simulink model "EKFSim"  (R2020a)
settings: Solver=VariableStepAuto  StartTime=0.0  StopTime=37500  RelTol=1e-3
undefined symbols (not defined in the file or in its folder): sigbuilder_block
libraries: fl_lib x14, nesl_utility x14
settings Model: Creator=WL  LastModifiedBy=Marvin
settings DataIOCC: ReturnWorkspaceOutputs=off
settings DebuggingCC: ArithmeticOperatorsInVariantConditions=warning
settings SFSimCC: SimUseLocalCustomCode=off  CustomCodeUndefinedFunction=UseInterfaceOnly
settings RTWCC: RTWUseLocalCustomCode=off
settings CodeAppCC: StateflowObjectComments=on

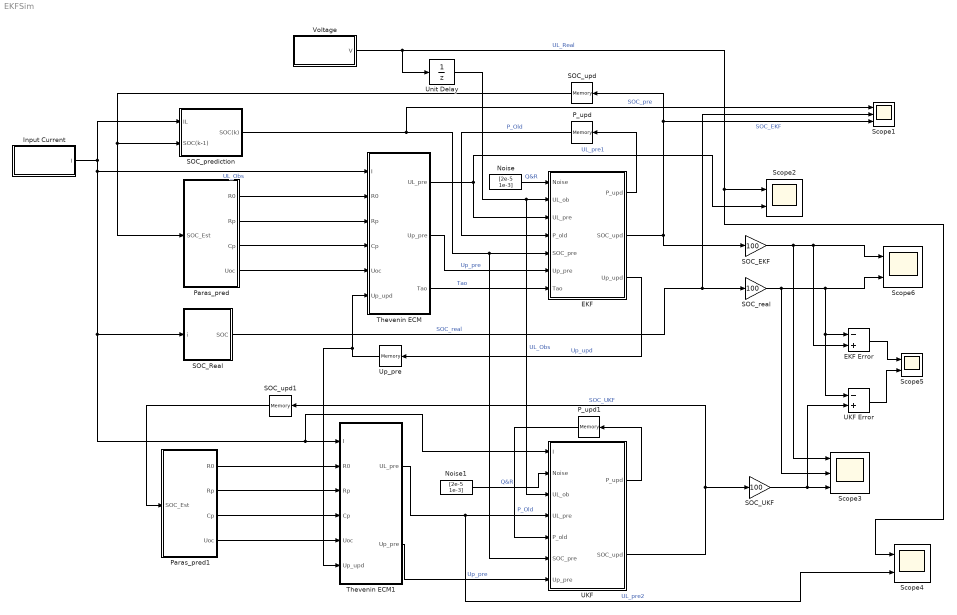
== system EKFSim ==
  EKF : MATLAB Function  TreatAsAtomicUnit=on
  EKF Error : Sum  Inputs=-+
  Input Current : Subsystem  Tag=STV Subsys  LoadFcn=sigbuilder_block('load');  StartFcn=sigbuilder_block('start');  StopFcn=sigbuilder_block('stop');  ClipboardFcn=sigbuilder_block('clipboard');  mask(Sigbuilder block){tuvar=[0:10]}
      mask help: Simulink:masks:SigbuilderBlock_MD
      mask init:
      | if ~strcmp(get_param(bdroot(gcbh),'SimulationStatus'),'stopped') tuvar = sigbuilder_block('maskInit'); end
      settings: CopyFcn=sigbuilder_block('copy');  DeleteFcn=sigbuilder_block('delete');  ModelCloseFcn=sigbuilder_block('modelClose');  PreSaveFcn=sigbuilder_block('preSave');  PauseFcn=sigbuilder_block('pause');  ContinueFcn=sigbuilder_block('continue');  NameChangeFcn=sigbuilder_block('namechange');  OpenFcn=sigbuilder_block('open',[6 51 1012.5 460.5 ]);  CloseFcn=sigbuilder_block('close');
      mask Display: plot(0, 0, 100, 100,[2, 2, 32, 32, 2], [68, 8, 8, 68, 68],[32, 2], [38, 38], [32, 19, 2],[53, 60, 44], [32, 17, 17, 2],[16, 16, 31, 31]);txt = getActiveGroup(gcbh);text(2, 100, txt,'verticalAlignment', 'top');
  Noise : Constant  Value=[2e-5 1e-3]
  Noise1 : Constant  Value=[2e-5 1e-3]
  P_upd : Memory  InitialCondition=[0.02 0 0 0.01]  InheritSampleTime=on  LinearizeAsDelay=on
  P_upd1 : Memory  InitialCondition=[1e-6 1e-6]  InheritSampleTime=on  LinearizeAsDelay=on
  Paras_pred : Subsystem
  Paras_pred1 : Subsystem
  SOC_EKF : Gain  Gain=100
  SOC_Real : Subsystem
  SOC_UKF : Gain  Gain=100
  SOC_prediction : Subsystem
  SOC_real : Gain  Gain=100
  SOC_upd : Memory  InitialCondition=1  InheritSampleTime=on  LinearizeAsDelay=on
  SOC_upd1 : Memory  InitialCondition=1  InheritSampleTime=on  LinearizeAsDelay=on
  Scope1 : Scope  NumInputPorts=3
  Scope{2,4..6} (4 alike) : Scope  NumInputPorts=2
  Scope3 : Scope  NumInputPorts=3
  Thevenin ECM : Subsystem
  Thevenin ECM1 : Subsystem
  UKF : MATLAB Function  TreatAsAtomicUnit=on
  UKF Error : Sum  Inputs=-+
  Unit Delay : UnitDelay  InitialCondition=4.1912  SampleTime=0.1  HasFrameUpgradeWarning=on
  Up_pre : Memory  InheritSampleTime=on  LinearizeAsDelay=on
  "Voltage " : Subsystem  Tag=STV Subsys  LoadFcn=sigbuilder_block('load');  StartFcn=sigbuilder_block('start');  StopFcn=sigbuilder_block('stop');  ClipboardFcn=sigbuilder_block('clipboard');  mask(Sigbuilder block){tuvar=[0:10]}
      mask help: Simulink:masks:SigbuilderBlock_MD
      mask init:
      | if ~strcmp(get_param(bdroot(gcbh),'SimulationStatus'),'stopped') tuvar = sigbuilder_block('maskInit'); end
      settings: CopyFcn=sigbuilder_block('copy');  DeleteFcn=sigbuilder_block('delete');  ModelCloseFcn=sigbuilder_block('modelClose');  PreSaveFcn=sigbuilder_block('preSave');  PauseFcn=sigbuilder_block('pause');  ContinueFcn=sigbuilder_block('continue');  NameChangeFcn=sigbuilder_block('namechange');  OpenFcn=sigbuilder_block('open',[6 51 1012.5 460.5 ]);  CloseFcn=sigbuilder_block('close');
      mask Display: plot(0, 0, 100, 100,[2, 2, 32, 32, 2], [68, 8, 8, 68, 68],[32, 2], [38, 38], [32, 19, 2],[53, 60, 44], [32, 17, 17, 2],[16, 16, 31, 31]);txt = getActiveGroup(gcbh);text(2, 100, txt,'verticalAlignment', 'top');
  wires:
  Paras_pred/4(Uoc) -> Thevenin ECM/5(Uoc)
  Paras_pred/1(R0) -> Thevenin ECM/2(R0)
  Paras_pred/3(Cp) -> Thevenin ECM/4(Cp)
  Paras_pred/2(Rp) -> Thevenin ECM/3(Rp)
  Thevenin ECM/1(UL_pre) -> Scope2/2, EKF/3(UL_pre)  "UL_pre1"
  "Voltage "/1(V) -> Unit Delay/1, Scope2/1, Scope4/1  "UL_Real"
  Thevenin ECM/2(Up_pre) -> EKF/6(Up_pre)  "Up_pre"
  Noise/1 -> EKF/1(Noise)  "Q&R"
  SOC_prediction/1(SOC(k)) -> Scope1/1, EKF/5(SOC_pre), UKF/6(SOC_pre)  "SOC_pre"
  P_upd/1 -> EKF/4(P_old)  "P_Old"
  SOC_upd/1 -> Paras_pred/1(SOC_Est), SOC_prediction/2(SOC(k-1))
  EKF/1(P_upd) -> P_upd/1
  Thevenin ECM/3(Tao) -> EKF/7(Tao)  "Tao"
  EKF/3(Up_upd) -> Up_pre/1  "Up_upd"
  Up_pre/1 -> Thevenin ECM1/6(Up_upd), Thevenin ECM/6(Up_upd)
  EKF/2(SOC_upd) -> SOC_EKF/1, Scope1/3, SOC_upd/1  "SOC_EKF"
  Unit Delay/1 -> UKF/3(UL_ob), EKF/2(UL_ob)  "UL_Obs"
  EKF Error/1 -> Scope5/1
  Noise1/1 -> UKF/2(Noise)  "Q&R"
  UKF/1(P_upd) -> P_upd1/1
  P_upd1/1 -> UKF/5(P_old)  "P_Old"
  Thevenin ECM1/1(UL_pre) -> Scope4/2, UKF/4(UL_pre)  "UL_pre2"
  Thevenin ECM1/2(Up_pre) -> UKF/7(Up_pre)  "Up_pre"
  UKF/2(SOC_upd) -> SOC_UKF/1, SOC_upd1/1  "SOC_UKF"
  Paras_pred1/1(R0) -> Thevenin ECM1/2(R0)
  Paras_pred1/2(Rp) -> Thevenin ECM1/3(Rp)
  Paras_pred1/3(Cp) -> Thevenin ECM1/4(Cp)
  Paras_pred1/4(Uoc) -> Thevenin ECM1/5(Uoc)
  SOC_upd1/1 -> Paras_pred1/1(SOC_Est)
  Input Current/1(I) -> SOC_Real/1(i), UKF/1(I), Thevenin ECM1/1(I), Thevenin ECM/1(I), SOC_prediction/1(IL)  "UL_Obs"
  SOC_Real/1(SOC) -> Scope1/2, SOC_real/1  "SOC_real"
  SOC_EKF/1 -> Scope6/1, EKF Error/2, Scope3/1
  SOC_real/1 -> Scope3/2, Scope6/2, UKF Error/1, EKF Error/1
  SOC_UKF/1 -> UKF Error/2, Scope3/3
  UKF Error/1 -> Scope5/2

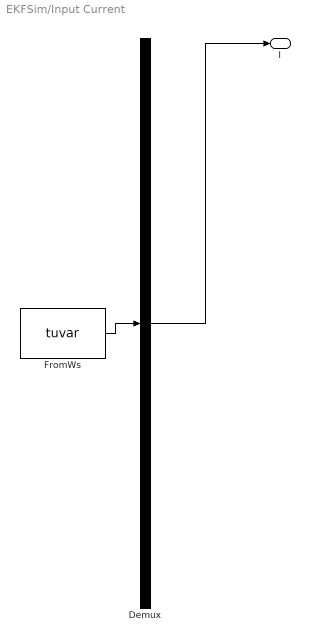
== system EKFSim/Input Current ==
  Demux : Demux  Tag=STV Demux  Outputs=1
      settings: DisplayOption=none
  FromWs : FromWorkspace  Tag=STV FromWs  VariableName=tuvar
      SigBuilderData=|
      | common.afterFinalStr = 'Extrapolate'
      | common.sampleTime = 0
      | dataSet.timeRange = [0 37520]
      | dataSet.name = 'Sheet1'
      | sbobj.Name = 'Signal Builder'
      | sbobj.Groups.Name = 'Sheet1'
      | sbobj.Groups.Signals.Name = 'I'
      | sbobj.Groups.Signals.XData = [0 1.01353925251 2.02707850502 3.04061775753 8.33038044522 13.6201431329 18.9099058206 24.1996685083 30.9141105575 35.6042291656 40.2943477737 44.9844663818 ... (4125 elements, 1x4125)]
      | sbobj.Groups.Signals.YData = [0.089857 0.0908255381097 0.0917940762194 0.0927626143291 0.0978175115535 0.0992265626287 0.0989541398502 0.0981051025856 0.1 0.0879771034309 0.0809245842985 0.0814437804285 ... (4125 elements, 1x4125)]
      | sbobj.Groups.TimeRange = [0 37520]
  I : Outport  VectorParamsAs1DForOutWhenUnconnected=off
  wires:
  Demux/1 -> I/1
  FromWs/1 -> Demux/1

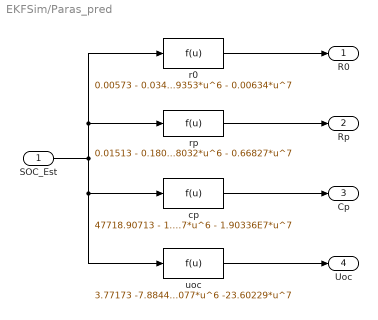
== system EKFSim/Paras_pred ==
  SOC_Est : Inport
  cp : Fcn  Expr=47718.90713 - 1.00583E6*u^1 + 9.2653E6*u^2 - 3.91088E7*u^3 + 8.85892E7*u^4 - 1.11014E8*u^5 + 7.22811E7*u^6 - 1.90336E7*u^7
  r0 : Fcn  Expr=0.00573 - 0.03427*u^1 + 0.1455*u^2 - 0.32647*u^3 + 0.41465*u^4 - 0.28992*u^5 + 0.09353*u^6 - 0.00634*u^7
  rp : Fcn  Expr=0.01513 - 0.18008*u^1 + 1.05147*u^2 - 3.27616*u^3 + 5.79793*u^4 - 5.81819*u^5 + 3.08032*u^6 - 0.66827*u^7
  uoc : Fcn  Expr=3.77173 -7.88447*u^1 + 60.21383*u^2 -200.15462*u^3 + 345.34531*u^4 - 314.92282*u^5 + 141.34077*u^6 -23.60229*u^7
  R0 : Outport  VectorParamsAs1DForOutWhenUnconnected=off
  Rp : Outport  Port=2  VectorParamsAs1DForOutWhenUnconnected=off
  Cp : Outport  Port=3  VectorParamsAs1DForOutWhenUnconnected=off
  Uoc : Outport  Port=4  VectorParamsAs1DForOutWhenUnconnected=off
  wires:
  cp/1 -> Cp/1
  rp/1 -> Rp/1
  uoc/1 -> Uoc/1
  r0/1 -> R0/1
  SOC_Est/1 -> uoc/1, cp/1, rp/1, r0/1

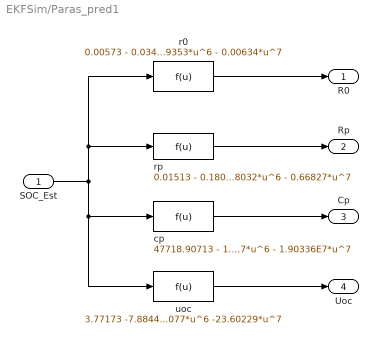
== system EKFSim/Paras_pred1 ==
  SOC_Est : Inport
  cp : Fcn  Expr=47718.90713 - 1.00583E6*u^1 + 9.2653E6*u^2 - 3.91088E7*u^3 + 8.85892E7*u^4 - 1.11014E8*u^5 + 7.22811E7*u^6 - 1.90336E7*u^7
  r0 : Fcn  Expr=0.00573 - 0.03427*u^1 + 0.1455*u^2 - 0.32647*u^3 + 0.41465*u^4 - 0.28992*u^5 + 0.09353*u^6 - 0.00634*u^7
  rp : Fcn  Expr=0.01513 - 0.18008*u^1 + 1.05147*u^2 - 3.27616*u^3 + 5.79793*u^4 - 5.81819*u^5 + 3.08032*u^6 - 0.66827*u^7
  uoc : Fcn  Expr=3.77173 -7.88447*u^1 + 60.21383*u^2 -200.15462*u^3 + 345.34531*u^4 - 314.92282*u^5 + 141.34077*u^6 -23.60229*u^7
  R0 : Outport  VectorParamsAs1DForOutWhenUnconnected=off
  Rp : Outport  Port=2  VectorParamsAs1DForOutWhenUnconnected=off
  Cp : Outport  Port=3  VectorParamsAs1DForOutWhenUnconnected=off
  Uoc : Outport  Port=4  VectorParamsAs1DForOutWhenUnconnected=off
  wires:
  cp/1 -> Cp/1
  rp/1 -> Rp/1
  uoc/1 -> Uoc/1
  SOC_Est/1 -> uoc/1, cp/1, r0/1, rp/1
  r0/1 -> R0/1

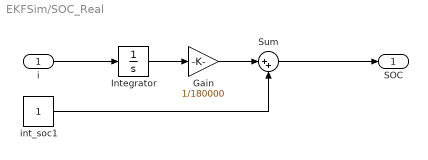
== system EKFSim/SOC_Real ==
  i : Inport
  Gain : Gain  Gain=1/180000
  Integrator : Integrator
  Sum : Sum  Inputs=|++
  int_soc1 : Constant
  SOC : Outport  VectorParamsAs1DForOutWhenUnconnected=off
  wires:
  Gain/1 -> Sum/1
  Integrator/1 -> Gain/1
  int_soc1/1 -> Sum/2
  i/1 -> Integrator/1
  Sum/1 -> SOC/1

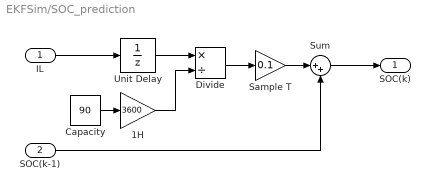
== system EKFSim/SOC_prediction ==
  IL : Inport
  SOC(k-1) : Inport  Port=2
  1H : Gain  Gain=3600
  Capacity : Constant  Value=90
  Divide : Product  Inputs=*/
  Sample T : Gain  Gain=0.1
  Sum : Sum  Inputs=|++
  Unit Delay : UnitDelay  SampleTime=0.15  HasFrameUpgradeWarning=on
  SOC(k) : Outport  VectorParamsAs1DForOutWhenUnconnected=off
  wires:
  Sample T/1 -> Sum/1
  Unit Delay/1 -> Divide/1
  SOC(k-1)/1 -> Sum/2
  IL/1 -> Unit Delay/1
  Sum/1 -> SOC(k)/1
  Capacity/1 -> 1H/1
  1H/1 -> Divide/2
  Divide/1 -> Sample T/1

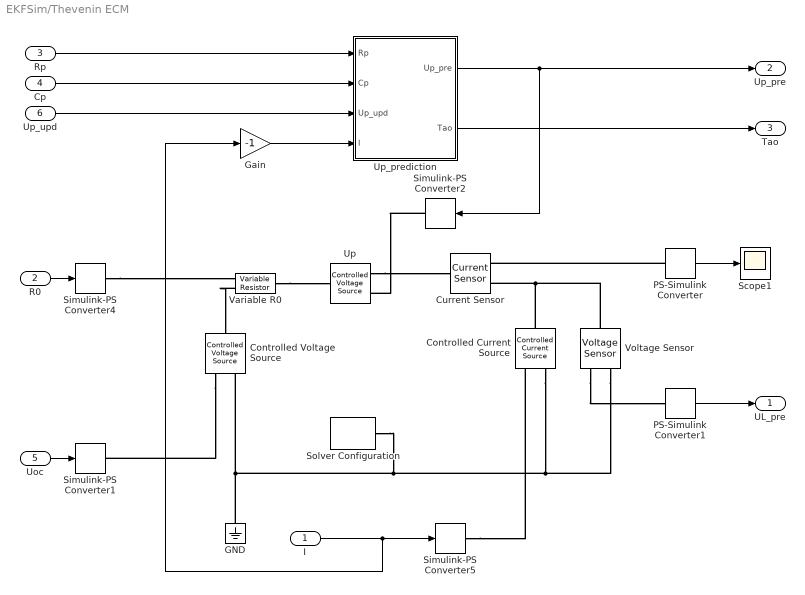
== system EKFSim/Thevenin ECM ==
  I : Inport
  R0 : Inport  Port=2
  Rp : Inport  Port=3
  Cp : Inport  Port=4
  Uoc : Inport  Port=5
  Up_upd : Inport  Port=6
  Controlled Current Source : fl_lib/Electrical/Electrical Sources/Controlled Current Source
  Controlled Voltage Source : fl_lib/Electrical/Electrical Sources/Controlled Voltage Source
  Current Sensor : fl_lib/Electrical/Electrical Sensors/Current Sensor
  GND : fl_lib/Electrical/Electrical Elements/Electrical Reference
  Gain : Gain  Gain=-1
  PS-Simulink Converter : nesl_utility/PS-Simulink Converter  PhysicalDomain=network_engine_domain  SubClassName=ps_output  LeftPortType=input  RightPortType=output  PseudoPeriodic=off  Frequencies=[]  Unit=A  AffineConversion=off
  PS-Simulink Converter1 : nesl_utility/PS-Simulink Converter  PhysicalDomain=network_engine_domain  SubClassName=ps_output  LeftPortType=input  RightPortType=output  PseudoPeriodic=off  Frequencies=[]  Unit=V  AffineConversion=off
  Scope1 : Scope
  Simulink-PS Converter{1..2,4..5} (4 alike) : nesl_utility/Simulink-PS Converter  PhysicalDomain=network_engine_domain  SubClassName=ps_input  LeftPortType=input  RightPortType=output  PseudoPeriodic=off  Frequencies=[]  NoiseDistribution=none  NoiseParameters=[]  Unit=1  AffineConversion=off  FilteringAndDerivatives=zero  SimscapeFilterOrder=1  InputFilterTimeConstant=0.001  UdotUserProvided=0
  Solver Configuration : nesl_utility/Solver Configuration  PhysicalDomain=network_engine_domain  SubClassName=solver  LeftPortType=input  RightPortType=generic  Tones=[]  Harmonics=[]  SimulateNoise=off  Profile=off  UseLocalSampling=off  EnableSwitchedLinearOptims=on  FrequencyDomain=off  UseCCode=off  RelTol=0.001  AbsTol=1e-06  MinStep=1e-09  ToWorkspace=off  RevertToSquareIcSolve=off  NumHomotopyIterations=100  PhasorMode=off  PhasorModeNumHarmonics=1  DoDC=off  ResidualTolerance=1e-09  UseLocalSolver=off  LocalSolverChoice=NE_BACKWARD_EULER_ADVANCER  LocalSolverSampleTime=0.001  DoFixedCost=off  MaxNonlinIter=3  MaxModeIter=2  LinearAlgebra=Sparse  EquationFormulation=NE_TIME_EF  DelaysMemoryBudget=1024  AutomaticFiltering=on  FilteringTimeConstant=0.001  PartitionStorageMethod=AS_NEEDED  PartitionMemoryBudget=1024  PartitionMethod=FAST
  Up : fl_lib/Electrical/Electrical Sources/Controlled Voltage Source
  Up_prediction : MATLAB Function  TreatAsAtomicUnit=on
  Variable R0 : fl_lib/Electrical/Electrical Elements/Variable Resistor  Rmin=0 Ohm  i_specify=off  i_priority=None  i=0 A  i_nominal_specify=off  i_nominal_unit=A  i_nominal_value=1  v_specify=off  v_priority=None  v=0 V  v_nominal_specify=off  v_nominal_unit=V  v_nominal_value=1
  Voltage Sensor : fl_lib/Electrical/Electrical Sensors/Voltage Sensor
  UL_pre : Outport  VectorParamsAs1DForOutWhenUnconnected=off
  Up_pre : Outport  Port=2  VectorParamsAs1DForOutWhenUnconnected=off
  Tao : Outport  Port=3  VectorParamsAs1DForOutWhenUnconnected=off
  wires:
  PS-Simulink Converter1/1 -> UL_pre/1
  Uoc/1 -> Simulink-PS Converter1/1
  Cp/1 -> Up_prediction/2(Cp)
  Rp/1 -> Up_prediction/1(Rp)
  R0/1 -> Simulink-PS Converter4/1
  I/1 -> Gain/1, Simulink-PS Converter5/1
  Up_prediction/1(Up_pre) -> Simulink-PS Converter2/1, Up_pre/1
  Up_upd/1 -> Up_prediction/3(Up_upd)
  Up_prediction/2(Tao) -> Tao/1
  Gain/1 -> Up_prediction/4(I)
  PS-Simulink Converter/1 -> Scope1/1
  connections:
  Variable R0/LConn2 -- Controlled Voltage Source/LConn1
  Controlled Current Source/LConn1 -- Voltage Sensor/LConn1 -- Current Sensor/RConn2
  Voltage Sensor/RConn2 -- Controlled Current Source/RConn2 -- Solver Configuration/RConn1 -- Controlled Voltage Source/RConn2 -- GND/LConn1
  PS-Simulink Converter/LConn1 -- Current Sensor/RConn1
  Voltage Sensor/RConn1 -- PS-Simulink Converter1/LConn1
  Controlled Voltage Source/RConn1 -- Simulink-PS Converter1/RConn1
  Simulink-PS Converter5/RConn1 -- Controlled Current Source/RConn1
  Simulink-PS Converter4/RConn1 -- Variable R0/LConn1
  Variable R0/RConn1 -- Up/LConn1
  Up/RConn2 -- Current Sensor/LConn1
  Simulink-PS Converter2/RConn1 -- Up/RConn1

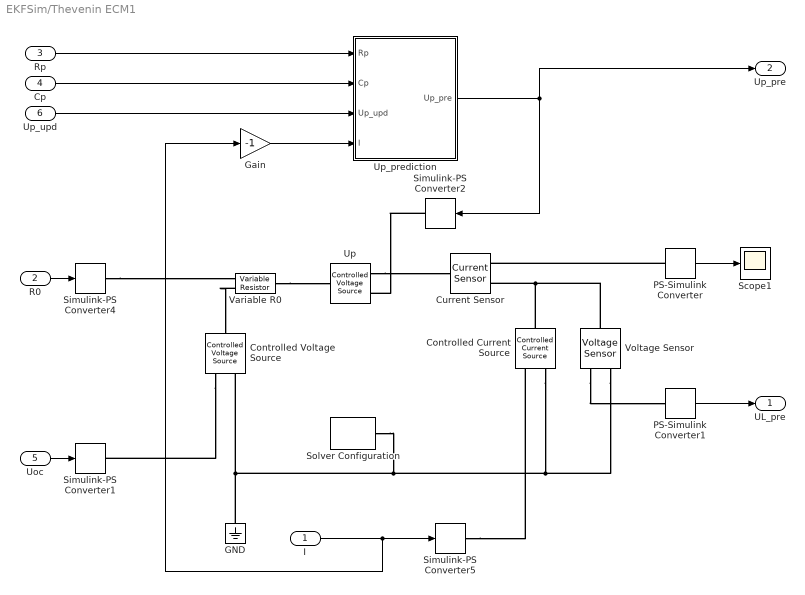
== system EKFSim/Thevenin ECM1 ==
  I : Inport
  R0 : Inport  Port=2
  Rp : Inport  Port=3
  Cp : Inport  Port=4
  Uoc : Inport  Port=5
  Up_upd : Inport  Port=6
  Controlled Current Source : fl_lib/Electrical/Electrical Sources/Controlled Current Source
  Controlled Voltage Source : fl_lib/Electrical/Electrical Sources/Controlled Voltage Source
  Current Sensor : fl_lib/Electrical/Electrical Sensors/Current Sensor
  GND : fl_lib/Electrical/Electrical Elements/Electrical Reference
  Gain : Gain  Gain=-1
  PS-Simulink Converter : nesl_utility/PS-Simulink Converter  PhysicalDomain=network_engine_domain  SubClassName=ps_output  LeftPortType=input  RightPortType=output  PseudoPeriodic=off  Frequencies=[]  Unit=A  AffineConversion=off
  PS-Simulink Converter1 : nesl_utility/PS-Simulink Converter  PhysicalDomain=network_engine_domain  SubClassName=ps_output  LeftPortType=input  RightPortType=output  PseudoPeriodic=off  Frequencies=[]  Unit=V  AffineConversion=off
  Scope1 : Scope
  Simulink-PS Converter{1..2,4..5} (4 alike) : nesl_utility/Simulink-PS Converter  PhysicalDomain=network_engine_domain  SubClassName=ps_input  LeftPortType=input  RightPortType=output  PseudoPeriodic=off  Frequencies=[]  NoiseDistribution=none  NoiseParameters=[]  Unit=1  AffineConversion=off  FilteringAndDerivatives=zero  SimscapeFilterOrder=1  InputFilterTimeConstant=0.001  UdotUserProvided=0
  Solver Configuration : nesl_utility/Solver Configuration  PhysicalDomain=network_engine_domain  SubClassName=solver  LeftPortType=input  RightPortType=generic  Tones=[]  Harmonics=[]  SimulateNoise=off  Profile=off  UseLocalSampling=off  EnableSwitchedLinearOptims=on  FrequencyDomain=off  UseCCode=off  RelTol=0.001  AbsTol=1e-06  MinStep=1e-09  ToWorkspace=off  RevertToSquareIcSolve=off  NumHomotopyIterations=100  PhasorMode=off  PhasorModeNumHarmonics=1  DoDC=off  ResidualTolerance=1e-09  UseLocalSolver=off  LocalSolverChoice=NE_BACKWARD_EULER_ADVANCER  LocalSolverSampleTime=0.001  DoFixedCost=off  MaxNonlinIter=3  MaxModeIter=2  LinearAlgebra=Sparse  EquationFormulation=NE_TIME_EF  DelaysMemoryBudget=1024  AutomaticFiltering=on  FilteringTimeConstant=0.001  PartitionStorageMethod=AS_NEEDED  PartitionMemoryBudget=1024  PartitionMethod=FAST
  Up : fl_lib/Electrical/Electrical Sources/Controlled Voltage Source
  Up_prediction : MATLAB Function  TreatAsAtomicUnit=on
  Variable R0 : fl_lib/Electrical/Electrical Elements/Variable Resistor  Rmin=0 Ohm  i_specify=off  i_priority=None  i=0 A  i_nominal_specify=off  i_nominal_unit=A  i_nominal_value=1  v_specify=off  v_priority=None  v=0 V  v_nominal_specify=off  v_nominal_unit=V  v_nominal_value=1
  Voltage Sensor : fl_lib/Electrical/Electrical Sensors/Voltage Sensor
  UL_pre : Outport  VectorParamsAs1DForOutWhenUnconnected=off
  Up_pre : Outport  Port=2  VectorParamsAs1DForOutWhenUnconnected=off
  wires:
  PS-Simulink Converter1/1 -> UL_pre/1
  Uoc/1 -> Simulink-PS Converter1/1
  Cp/1 -> Up_prediction/2(Cp)
  Rp/1 -> Up_prediction/1(Rp)
  R0/1 -> Simulink-PS Converter4/1
  I/1 -> Gain/1, Simulink-PS Converter5/1
  Up_prediction/1(Up_pre) -> Up_pre/1, Simulink-PS Converter2/1
  Up_upd/1 -> Up_prediction/3(Up_upd)
  Gain/1 -> Up_prediction/4(I)
  PS-Simulink Converter/1 -> Scope1/1
  connections:
  Variable R0/LConn2 -- Controlled Voltage Source/LConn1
  Controlled Current Source/LConn1 -- Voltage Sensor/LConn1 -- Current Sensor/RConn2
  Voltage Sensor/RConn2 -- Controlled Current Source/RConn2 -- Solver Configuration/RConn1 -- Controlled Voltage Source/RConn2 -- GND/LConn1
  PS-Simulink Converter/LConn1 -- Current Sensor/RConn1
  Voltage Sensor/RConn1 -- PS-Simulink Converter1/LConn1
  Controlled Voltage Source/RConn1 -- Simulink-PS Converter1/RConn1
  Simulink-PS Converter5/RConn1 -- Controlled Current Source/RConn1
  Simulink-PS Converter4/RConn1 -- Variable R0/LConn1
  Variable R0/RConn1 -- Up/LConn1
  Up/RConn2 -- Current Sensor/LConn1
  Simulink-PS Converter2/RConn1 -- Up/RConn1

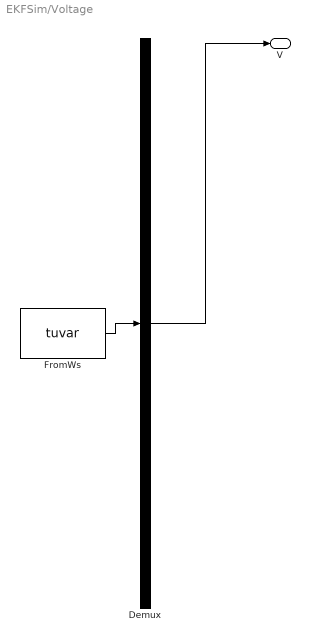
== system EKFSim/Voltage  ==
  Demux : Demux  Tag=STV Demux  Outputs=1
      settings: DisplayOption=none
  FromWs : FromWorkspace  Tag=STV FromWs  VariableName=tuvar
      SigBuilderData=|
      | common.afterFinalStr = 'Extrapolate'
      | common.sampleTime = 0
      | dataSet.timeRange = [0 37520]
      | dataSet.name = 'Sheet1'
      | sbobj.Name = 'Signal Builder'
      | sbobj.Groups.Name = 'Sheet1'
      | sbobj.Groups.Signals.Name = 'V'
      | sbobj.Groups.Signals.XData = [0 1.01353925251 2.02707850502 3.04061775753 8.33038044522 13.6201431329 18.9099058206 24.1996685083 30.9141105575 35.6042291656 40.2943477737 44.9844663818 ... (4125 elements, 1x4125)]
      | sbobj.Groups.Signals.YData = [4.19119264765 4.19120586861 4.19121888844 4.19123172277 4.19129665352 4.19132225272 4.19132889262 4.1913282962 4.19131131025 4.19124102157 4.1911747464 4.19118346146 ... (4125 elements, 1x4125)]
      | sbobj.Groups.TimeRange = [0 37520]
  V : Outport  VectorParamsAs1DForOutWhenUnconnected=off
  wires:
  Demux/1 -> V/1
  FromWs/1 -> Demux/1

== matlab function EKFSim/Thevenin ECM/Up_prediction ==
  data: Rp input; Up_pre output; Cp input; Up_upd input; Tao output; I input
function [Up_pre, Tao] = fcn(Rp, Cp,Up_upd,I)
Tao = Rp*Cp;
Up_pre=exp(-0.1/Tao)*Up_upd+Rp*(1-exp(-0.1/Tao))*I;

== matlab function EKFSim/EKF ==
  data: P_upd output; Noise input; UL_ob input; UL_pre input; P_old input; SOC_pre input; Up_pre input; Tao input; SOC_upd output; Up_upd output
function [P_upd,SOC_upd,Up_upd] = EKF(Noise, UL_ob, UL_pre, P_old, SOC_pre, Up_pre, Tao)
Q = Noise(1);   
R = Noise(2);   

%% --------------A Matrix, state transition----------
A1 = 1;
A2 = exp(-0.05/Tao);
A = [A1 0;0 A2];

P_last = [P_old(1) P_old(2);P_old(3) P_old(4)];
P_pre=A*P_last*A'+ [Q 0;0 Q];  
%% --------------C matrix-------------
C1 = 2575090.4551015184 -6666328.439687796*SOC_pre + 7512344.5273519205*SOC_pre^2 -4813117.931864428*SOC_pre^3 + 1917539.5659157163*SOC_pre^4 -486428.46157733985*SOC_pre^5 + 76726.2212424136*SOC_pre^6 -6880.127940314166*SOC_pre^7 + 268.529995224067*SOC_pre^8;
C = [C1 -1];
%% --------------Update--------------
X_pre = [SOC_pre;Up_pre];
K = P_pre*C'*(C*P_pre*C'+ R)^(-1);     
X_upd = X_pre + K*(UL_ob-UL_pre);     
P_update = P_pre - K*C*P_pre;
%% --------------Output--------------
SOC_upd = X_upd(1);
Up_upd = X_upd(2);
P_upd = [P_update(1,1) P_update(1,2) P_update(2,1) P_update(2,2)];

== matlab function EKFSim/UKF ==
  data: I input; P_upd output; Noise input; UL_ob input; UL_pre input; P_old input; SOC_pre input; Up_pre input; SOC_upd output
function [P_upd,SOC_upd] = UKF(I, Noise, UL_ob, UL_pre, P_old, SOC_pre, Up_pre)
Q = Noise(1);   
R = Noise(2); 
n=1;  
alp=0.04;
beta=2;                                                       
lamda=1.5;
%% ---------------Weight determination---------------
 Wm=[lamda/(n+lamda),0.5/(n+lamda)+zeros(1,2*n)];                               
 Wc=Wm;
 Wc(1)=Wc(1)+(1-alp^2+beta);

%% --------------Initialize--------------     
X_pre = [SOC_pre-0.009; Up_pre];
Xsigma=X_pre;
pk=sqrt((n+lamda)*P_old);

%% ---------------Determine sigma sampling point------------
sigma1 = Xsigma+pk;
sigma2 = Xsigma-pk;
sigma=[Xsigma sigma1 sigma2];

%% -------------System state prediction equation----------------
sxk=0;     
for ks=1:2*n+1
    sigma(ks)=sigma(ks)-(I*0.1)/(2.7*3600);
    sxk=Wm(ks)*sigma(ks)+sxk;      
end

spk=0;    
for kp=1:2*n+1
    spk=Wc(kp)*(sigma(kp)-sxk)*(sigma(kp)-sxk)'+spk;  
end
spk=spk+Q;

%% ------Measurement Update--------
syk=0;     
for ky=1:2*n+1
    syk=syk+Wm(ky)*UL_pre;     
end

pyy=0;     
for kpy=1:2*n+1
    pyy=Wc(kpy)*(UL_pre-syk)*(UL_pre-syk)'+pyy;    
end
pyy=pyy+R;

%% --------------Error covariance--------------
pxy=0;     
for kxy=1:2*n+1
    pxy=Wc(kxy)*(sigma(kxy)-sxk)*(UL_pre-syk)'+pxy;  
end

%% ------------Kalman gain-----------
kgs=pxy/pyy; 

%% ------------State and error covariance matrix update------
X_upd=sxk+kgs*(UL_ob-syk);    
P_update=spk-kgs*pyy*kgs';          

%% --------------Output--------------
SOC_upd = X_upd;
P_upd = P_update;

== matlab function EKFSim/Thevenin ECM1/Up_prediction ==
  data: Rp input; Up_pre output; Cp input; Up_upd input; I input
function Up_pre  = fcn(Rp, Cp,Up_upd,I)
Tao = Rp*Cp;
Up_pre=exp(-0.1/Tao)*Up_upd+Rp*(1-exp(-0.1/Tao))*I;
